simulink model "Controle_Lab4_model_2012b"  (R2012b)
settings: Solver=ode45  StartTime=0.0  StopTime=6  RelTol=1e-3
values from neighbouring files (symbols this model uses):
  K = 0.02    [Controle_Lab4.m]    (also in Lab8.m = place(A,B,[-10 -12 -2]); Tarefa1.m)
  Kp = Kkp/K    (= 358.333333333)    [Controle_Lab4.m]    (also in Tarefa1.m = 300)
  KpInt = 0.9 * (T/L)    (= 6.45)    [Controle_Lab4.m]
  KpInt2 = 0.45 * Kcrit    (= 185.443883594)    [Controle_Lab4.m]
  L = 1.024 - Start    (= 0.024)    [Controle_Lab4.m]    (also in Tarefa1.m = 0.03)
  T = 1.196 - L - Start    (= 0.172)    [Controle_Lab4.m]    (also in Tarefa1.m = 0.18)
  Ti1 = L/0.3    (= 0.08)    [Controle_Lab4.m]
  Ti2 = (1/1.2) * Pcrit    (= 0.121767157116)    [Controle_Lab4.m]
settings Model: Creator=11104980  LastModifiedBy=11104980
settings DebuggingCC: FrameProcessingCompatibilityMsg=error
settings CodeAppCC: CustomSymbolStrType=$N$R$M_T
settings GRTTargetCC: CodeReplacementLibrary=C89/C90 (ANSI)

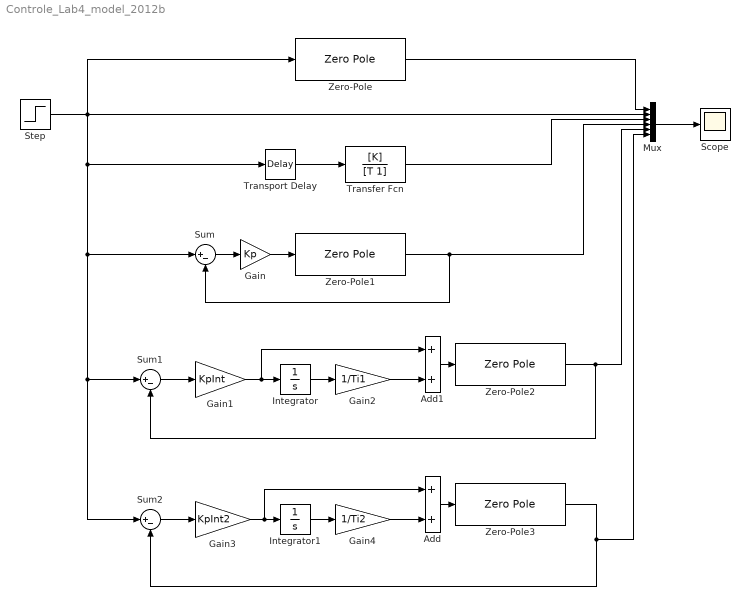
== system Controle_Lab4_model_2012b ==
  Add : Sum
  Add1 : Sum
  Gain : Gain  Gain=Kp
  Gain1 : Gain  Gain=KpInt
  Gain2 : Gain  Gain=1/Ti1
  Gain3 : Gain  Gain=KpInt2
  Gain4 : Gain  Gain=1/Ti2
  Integrator : Integrator
  Integrator1 : Integrator
  Mux : Mux  Inputs=6
  Scope : Scope
      settings: SaveName=y
  Step : Step  SampleTime=0
  Sum : Sum  Inputs=|+-
  Sum1 : Sum  Inputs=|+-
  Sum2 : Sum  Inputs=|+-
  Transfer Fcn : TransferFcn  Numerator=[K]  Denominator=[T 1]
  Transport Delay : TransportDelay  DelayTime=L
  Zero-Pole{,1..3} (4 alike) : ZeroPole  Zeros=[]  Poles=[-20 -25 -30]  Gain=[300]
  wires:
  Zero-Pole/1 -> Mux/1
  Mux/1 -> Scope/1
  Transport Delay/1 -> Transfer Fcn/1
  Transfer Fcn/1 -> Mux/3
  Zero-Pole2/1 -> Sum1/2, Mux/5
  Sum1/1 -> Gain1/1
  Gain1/1 -> Add1/1, Integrator/1
  Integrator/1 -> Gain2/1
  Sum/1 -> Gain/1
  Gain/1 -> Zero-Pole1/1
  Zero-Pole1/1 -> Sum/2, Mux/4
  Zero-Pole3/1 -> Sum2/2, Mux/6
  Sum2/1 -> Gain3/1
  Gain3/1 -> Add/1, Integrator1/1
  Integrator1/1 -> Gain4/1
  Step/1 -> Mux/2, Transport Delay/1, Sum/1, Sum1/1, Sum2/1, Zero-Pole/1
  Add/1 -> Zero-Pole3/1
  Gain4/1 -> Add/2
  Gain2/1 -> Add1/2
  Add1/1 -> Zero-Pole2/1
